simulink model "RP_DCE_new_kyvadlo_polynomial"  (R2014b)
settings: Solver=ode45  StartTime=0.0  StopTime=inf  RelTol=1e-3
values from neighbouring files (symbols this model uses):
  C_norm = C / 16    [glabatom_pokus.m]
undefined symbols (not defined in the file or in its folder): Humusoft, kkyv_rad, kram_rad, MF614
libraries: rtwinlib x2
settings Model: Creator=student  LastModifiedBy=student

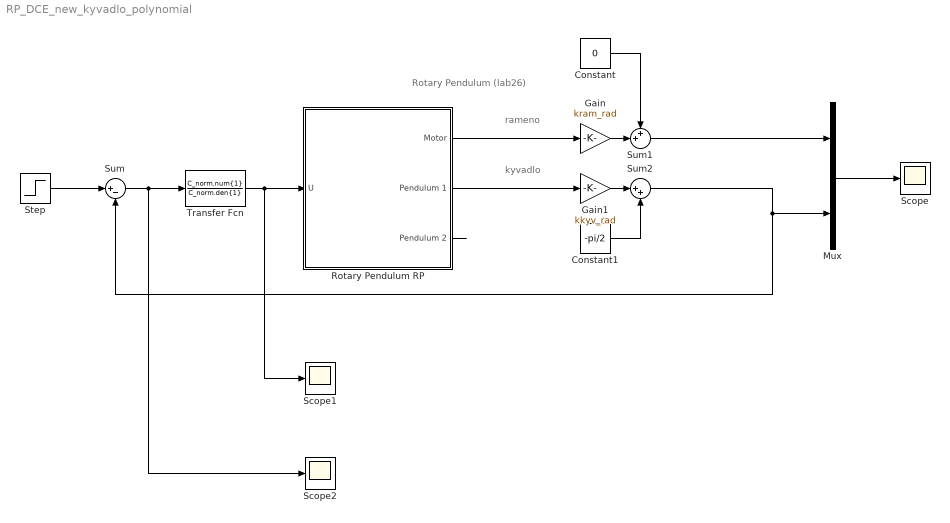
== system RP_DCE_new_kyvadlo_polynomial ==
  note: kyvadlo
  note: rameno
  note: Rotary Pendulum (lab26)
  Constant : Constant  Value=0
  Constant1 : Constant  Value=-pi/2
  Gain : Gain  Gain=kram_rad
  Gain1 : Gain  Gain=kkyv_rad
  Mux : Mux  Inputs=2
  "Rotary Pendulum RP " : Subsystem  mask(Rotary Pendulum RP in Laboratory K26){Ts=0.005, U_init=0, U_final=0}
      mask prompts: Ts "Sampling Time {Ts = 0.005 s; <0.02 ...0.001>}"; U_init "Initial Input Value {U_init = 0; <-1 ... 1>}"; U_final "Final Input Value {U_final = 0; <-1 ... 1>}"
      mask help: Rotary Pendulum RP in Laboratory K26 - Real Time Communication
      mask Help:
      | Rotary Pendulum in Laboratory K26 - Real Time Communication. <br><br>
      | 
      | This is a model of the Rotary Pendulum. The motor is rotate the mass with a pivot. Pendulum 1 is hung on the mass on the pivot and pendulum 2 is hugh on the pendulum 1. <br><br>
      | 
      | There are one input and three outputs in the model. The input is a volatage of the motor between -10 and 10 volts. Outputs are the real motor angle and the real angles of the pendulum 1 and pendulum 2. In Simulink, the signals are normalized to interval (-1; +1). <br><br>
      | 
      | You can set a samplig time and you can set an initial and a final value of the input voltage of the motor.
      mask Display:
      | % plot(-2,-1,2,1,[-1,-1,0.3,0.3,-1],[-0.8,-0.6,-0.6,-0.8,-0.8]);
      | % plot(-2,-1,2,1,[-0.8,-0.8,0,0,-0.8],[-0.6,0.8,0.8,-0.6,-0.6]);
      | % plot(-2,-1,2,1,[-0.8,-0.8,0.8,0.8,-0.8],[0.6,0.8,0.8,0.6,0.6]);
      | % plot(-2,-1,2,1,[-0.8,-0.6,-0.6,-0.4,-0.4,-0.2,-0.2,0,0],[0.8,0.6,0.8,0.6,0.8,0.6,0.8,0.6,0.8]);
      | % plot(-2,-1,2,1,[0.7,0.8,0.8,0.7,0.7],[0.8,0.8,0.2,0.2,0.8],[0.72,0.76,0.76,0.72,0.72],[0.78,0.78,0.22,0.22,0.78],[0.74,0.72,0.72,0.74,0.74],[0.76,0.76,0.24,0.24,0.76]);
      | image(imread('rotacni_kyvadlo_simulink.tif'))
  Scope : Scope
      settings: TimeRange=5  YMin=-3  YMax=3  SaveName=scopearray  MaxDataPoints=500000
  Scope1 : Scope
      settings: TimeRange=5  YMin=-80  YMax=60  SaveName=scopearray1  MaxDataPoints=500000
  Scope2 : Scope
      settings: TimeRange=5  YMin=-80  YMax=60  SaveName=scopearray2  MaxDataPoints=500000
  Step : Step  Time=0  After=-pi/2  SampleTime=0
  Sum : Sum  Inputs=|+-
  Sum1 : Sum  Inputs=++|
  Sum2 : Sum  Inputs=|++
  Transfer Fcn : TransferFcn  Numerator=C_norm.num{1}  Denominator=C_norm.den{1}
  wires:
  Mux/1 -> Scope/1
  "Rotary Pendulum RP "/1(Motor) -> Gain/1
  "Rotary Pendulum RP "/3(Pendulum 2) -> ?
  Sum/1 -> Scope2/1, Transfer Fcn/1
  Transfer Fcn/1 -> Scope1/1, "Rotary Pendulum RP "/1(U)
  Step/1 -> Sum/1
  Gain/1 -> Sum1/2
  Constant/1 -> Sum1/1
  Sum1/1 -> Mux/1
  "Rotary Pendulum RP "/2(Pendulum 1) -> Gain1/1
  Sum2/1 -> Sum/2, Mux/2
  Gain1/1 -> Sum2/1
  Constant1/1 -> Sum2/2

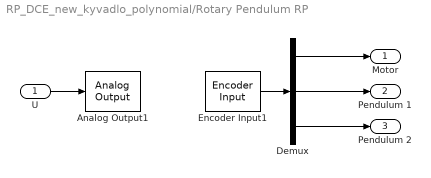
== system RP_DCE_new_kyvadlo_polynomial/Rotary Pendulum RP  ==
  U : Inport
  Analog Output1 : rtwinlib/Analog Output  SampleTime=Ts  MaxMissedTicks=1000  ShowMissedTicks=off  YieldWhenWaiting=on  DrvName=Humusoft/MF614  DrvAddress=4294967295  DrvOptions=0  Channels=1  RangeMode=2  VoltRange=1  InitialValue=[U_init]  FinalValue=[U_final]
      settings: AttributesFormatString=Humusoft\nMF614 [auto]
  Demux : Demux  Outputs=3
  Encoder Input1 : rtwinlib/Encoder Input  SampleTime=Ts  MaxMissedTicks=1000  ShowMissedTicks=off  YieldWhenWaiting=on  DrvName=Humusoft/MF614  DrvAddress=4294967295  DrvOptions=0  Channels=[2,4,1]  QuadMode=3  IndexPulse=3  InputFilter=Inf  DataType=1
      settings: AttributesFormatString=Humusoft\nMF614 [auto]
  Motor : Outport
  Pendulum 1 : Outport  Port=2
  Pendulum 2 : Outport  Port=3
  wires:
  Encoder Input1/1 -> Demux/1
  U/1 -> Analog Output1/1
  Demux/3 -> Pendulum 2/1
  Demux/1 -> Motor/1
  Demux/2 -> Pendulum 1/1
